simulink model "eg1"  (R2015a)
settings: Solver=ode45  StartTime=0.0  StopTime=200  RelTol=1e-3
settings Model: Creator=ayush  LastModifiedBy=ayush

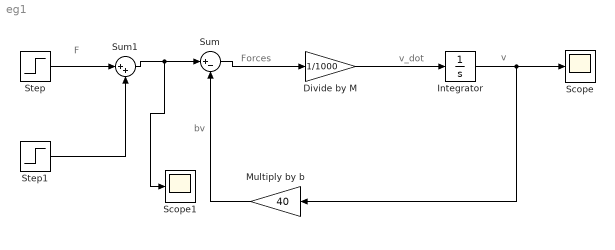
== system eg1 ==
  note: bv
  note: v
  note: v_dot
  note: Forces
  note: F
  Divide by M : Gain  Gain=1/1000
  Integrator : Integrator
  Multiply by b : Gain  Gain=40
  Scope : Scope
  Scope1 : Scope
  Step : Step  Time=0  After=400  SampleTime=0
  Step1 : Step  Time=100  After=-400  SampleTime=0
  Sum : Sum  Inputs=|+-
  Sum1 : Sum  Inputs=|++
  wires:
  Sum/1 -> Divide by M/1
  Divide by M/1 -> Integrator/1
  Integrator/1 -> Multiply by b/1, Scope/1
  Step/1 -> Sum1/1
  Multiply by b/1 -> Sum/2
  Sum1/1 -> Scope1/1, Sum/1
  Step1/1 -> Sum1/2
